simulink model "Motor_MapMdl_Ptbs_V1"  (R2018a)
settings: configuration reference "Config_Plant" (kept outside this file)
PreLoadFcn:
  | Motor_MapMdl_Ptbs_V1_BusInfo
model workspace (MAT data in the model file):
  mot.max_trq = 307
  mot.max_pwr = 124
  mot.spd = [0 500 1000 1500 2000 2500 3000 3500 3857.04487493 4000 4500 5000 5500 6000 6500 7000 7500 8000 8500 9000 9500 10000 10500 11000 11500 12000 12500]
  mot.trq = [307 307 307 307 307 307 307 307 307 296.028194151 263.136172579 236.822555321 215.29323211 197.352129434 182.171196401 169.158968086 157.881703547 148.014097075 139.307385483 131.568086289 124.643450169 118.41127766 112.772645391 107.646616055 102.9663284 98.676064717 94.7290221283]
  mot.trq_cp = [296.028194151 263.136172579 236.822555321 215.29323211 197.352129434 182.171196401 169.158968086 157.881703547 148.014097075 139.307385483 131.568086289 124.643450169 118.41127766 112.772645391 107.646616055 102.9663284 98.676064717 94.7290221283]
  mot.J = 0.02
  mot.damp = 0.0001
  mot.Tc = 0.0267
  mot.map.spdindex = [0 1000 2000 3000 3857 4000 5000 6000 7000 8000 9000 10000 11000 12000 12584]
  mot.map.trqindex = [10 25 50 75 100 125 150 175 200 225 250 275 300 307]
  mot.map.eff = [84  90  90  90  90  90  90  90  90  90  90  90  90  90  90; 84  90  93  95  95  95  96  95  95  95  95  93  93  93  93; 84  90  93  95  95  95  96  95  96  95  95  95  95  93  93; 84  90  93  95  95  95  96  96  96  95  95  95  95  93  93; 84  90  93  95  95  95  96  96  96  95  95  93  93  93  90; 84  88  90  93  93  95  95  96  95  95  95  93  93  93  90; 84  88  90  90  90  93  95  95  95  93  93  93  93  93  90; 84  88  90  90  90  90  93  93  93  93  93  93  93  93  90; 84  84  88  90  90  90  93  93  93  93  93  93  93  93  90; 84  84  88  90  90  90  90  93  93  93  93  93  93  93  90; 84  84  84  90  90  90  90  93  93  93  93  93  93  93  90; 84  84  84  88  90  90  90  93  93  93  93  93  93  93  90; 84  84  84  88  88  88  90  93  93  93  93  93  93  93  90; 84  84  84  88  88  88  90  93  93  93  93  93  93  93  90]
  mot.m = 30
  mot.Cp = 200
values from neighbouring files (symbols this model uses):
  mot = struct    [Motor_V1.m]
libraries: autolibmappedmotor x1
settings Model: Creator=IAEC Nishito  LastModifiedBy=E00026
settings ConfigSetRef: SourceLocation=Base Workspace

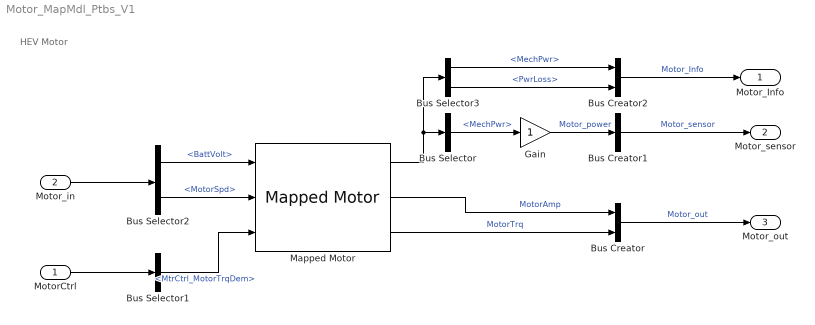
== system Motor_MapMdl_Ptbs_V1 ==
  note: HEV Motor
  MotorCtrl : Inport  OutDataTypeStr=Bus: MotorCtrl_Bus  SampleTime=0
      settings: AttributesFormatString=%<OutDataTypeStr>
  Motor_in : Inport  Port=2  OutDataTypeStr=Bus: Motor_in_Bus
      settings: AttributesFormatString=%<OutDataTypeStr>
  Bus Creator : BusCreator  Inputs=2  OutDataTypeStr=Bus: Motor_out_Bus
      settings: AttributesFormatString=%<OutDataTypeStr>
  Bus Creator1 : BusCreator  Inputs=1  OutDataTypeStr=Bus: Motor_sensor_Bus
      settings: AttributesFormatString=%<OutDataTypeStr>
  Bus Creator2 : BusCreator  Inputs=2  OutDataTypeStr=Bus: Motor_Info_out_Bus
      settings: AttributesFormatString=%<OutDataTypeStr>
  Bus Selector : BusSelector  OutputSignals=MechPwr
  Bus Selector1 : BusSelector  OutputSignals=MtrCtrl_MotorTrqDem
  Bus Selector2 : BusSelector  OutputSignals=BattVolt,MotorSpd
  Bus Selector3 : BusSelector  OutputSignals=MechPwr,PwrLoss
  Gain : Gain
  Mapped Motor : autolibmappedmotor/Mapped Motor  port_config=Speed  param_by=Maximum torque and power  w_t=[ 0 375 750 800 ]  T_t=[0.09 0.08 0.07 0]  torque_max=307  power_max=124e3  Tc=0.02  param_loss=Tabulated efficiency data  eff=100  w_eff=375  T_eff=0.08  Piron=0  Pbase=0  w_eff_bp=mot.map.spdindex.*pi/30  T_eff_bp=mot.map.trqindex  losses_table=[1 2;3 4]  efficiency_table=mot.map.eff'  J=5e-6  b=1e-5  omega_o=0  T_t_extended=[0 0.07 0.08 0.09 0.08 0.07 0]  w_t_extended=[-800 -750 -375 0 375 750 800]  KLossIron=0  KLossCopper=0  x_w_eff_vec=[-1317.7933984258 -1256.63706143592 -1151.91730631626 -1047.1975511966 -942.477796076938 -837.758040957278 -733.038285837618 -628.318530717959 -523.598775598299 -418.879020478639 -403.904095496528 -314.159265358979 -209.43951023932 -104.71975511966 0 104.71975511966 209.43951023932 314.159265358979 403.904095496528 418.879020478639 523.598775598299 628.318530717959 733.038285837618 837.758040957278 942.477796076938 1047.1975511966 1151.91730631626 1256.63706143592 1317.7933984258]  x_T_eff_vec=[-307 -300 -275 -250 -225 -200 -175 -150 -125 -100 -75 -50 -25 -10 10 25 50 75 100 125 150 175 200 225 250 275 300 307]  x_losses_mat=[44951.3970351912 43926.4466141933 40265.9093963439 36605.3721784944 32944.834960645 29284.2977427955 25623.7605249461 21963.2233070967 18302.6860892472 14642.1488713978 7439.15628143595 4959.4375209573 2479.71876047865 1464.21488713978 1317.7933984258 2306.13844724515 4612.27689449029 6918.41534173544 13177.933984258 16472.4174803225 19766.900976387 23061.3844724515 26355.867968516 29650.3514645805 32944.834960645 36239.3184567095 39533.801952774 40456.257331672;29037.7746776966 28375.675580811 26011.0359490768 23646.3963173425 21281.7566856083 18917.117053874 16552.4774221398 14187.8377904055 11823.1981586713 9458.558526937 7093.91889520275 4729.2792634685 2364.63963173425 1396.26340159546 1256.63706143592 2199.11485751285 4398.22971502571 6597.34457253856 8796.45943005141 10995.5742875643 13194.6891450771 15393.80400259 17592.9188601028 19792.0337176157 21991.1485751285 24190.2634326414 26389.3782901542 27005.1304502578;26617.9601212219 26011.0359490768 23843.449619987 21675.8632908973 19508.2769618076 17340.6906327178 15173.1043036281 13005.5179745384 10837.9316454486 8670.34531635892 4547.0419986168 3031.3613324112 2167.58632908973 1279.90811812918 1151.91730631626 2015.85528605345 2879.79326579064 4319.68989868596 8063.4211442138 10079.2764302672 12095.1317163207 14110.9870023741 16126.8422884276 18142.697574481 20158.5528605345 22174.4081465879 24190.2634326414 24754.7029127364;24198.1455647472 23646.3963173425 21675.8632908973 19705.3302644521 17734.7972380069 15764.2642115617 13793.7311851165 11823.1981586713 9852.66513222605 7882.13210578084 4133.67454419709 2755.78302946473 1970.53302644521 1163.55283466289 1047.1975511966 1832.59571459404 2617.99387799149 3926.99081698724 7330.38285837618 9162.97857297022 10995.5742875643 12828.1700021583 14660.7657167524 16493.3614313464 18325.9571459404 20158.5528605345 21991.1485751285 22504.2753752149;21778.3310082725 21281.7566856083 19508.2769618076 17734.7972380069 15961.3175142062 14187.8377904055 12414.3580666048 10640.8783428041 6200.51181629564 4960.40945303651 3720.30708977738 2480.20472651826 1240.10236325913 1047.1975511966 942.477796076938 1178.09724509617 2356.19449019234 3534.29173528851 4712.38898038468 5890.48622548085 9896.01685880784 11545.3530019425 13194.6891450771 14844.0252882118 16493.3614313464 18142.697574481 19792.0337176157 20253.8478376934;19358.5164517977 18917.117053874 17340.6906327178 15764.2642115617 14187.8377904055 12611.4113692493 11034.9849480932 9458.558526937 5511.56605892945 4409.25284714356 3306.93963535767 2204.62642357178 1102.31321178589 930.842267730309 837.758040957278 1047.1975511966 2094.39510239319 3141.59265358979 4188.79020478639 5235.98775598298 8796.45943005141 10262.5360017266 11728.6125734019 13194.6891450771 14660.7657167524 16126.8422884276 17592.9188601028 18003.4203001719;16938.701895323 16552.4774221398 15173.1043036281 13793.7311851165 12414.3580666048 11034.9849480932 9655.61182958152 5787.14436187593 4822.62030156327 3054.32619099008 2290.74464324256 1527.16309549504 964.524060312655 814.486984264021 733.038285837618 916.297857297022 1466.07657167524 2199.11485751286 2932.15314335048 4581.48928648511 5497.78714378213 8979.71900151082 10262.5360017266 11545.3530019425 12828.1700021583 14110.9870023741 15393.80400259 15752.9927626504;14518.8873388483 14187.8377904055 13005.5179745384 11823.1981586713 10640.8783428041 9458.558526937 8276.23871106988 4960.40945303651 3272.49234748937 2617.9938779915 1963.49540849362 1653.46981767884 826.734908839418 698.131700797732 628.318530717959 785.398163397447 1570.79632679489 1884.95559215388 2513.27412287184 3141.5926535898 4712.38898038468 7696.90200129499 8796.45943005141 9896.01685880784 10995.5742875643 12095.1317163207 13194.6891450771 13502.5652251289;17860.5360120753 17453.2925199433 15998.8514766147 14544.4104332861 13089.9693899575 7882.13210578084 6896.86559255823 4133.67454419709 3444.72878683091 2181.66156499292 1636.24617374469 1090.83078249646 545.415391248229 ...(+9284 chars)]  aMode=aMode
      settings: SourceProductName=Powertrain Blockset  SourceProductBaseCode=PW
  Motor_Info : Outport  OutDataTypeStr=Bus: Motor_Info_out_Bus
      settings: AttributesFormatString=%<OutDataTypeStr>
  Motor_sensor : Outport  Port=2  OutDataTypeStr=Bus: Motor_sensor_Bus
      settings: AttributesFormatString=%<OutDataTypeStr>
  Motor_out : Outport  Port=3  OutDataTypeStr=Bus: Motor_out_Bus
      settings: AttributesFormatString=%<OutDataTypeStr>
  wires:
  Mapped Motor/2 -> Bus Creator/1  "MotorAmp"
  Mapped Motor/1 -> Bus Selector3/1, Bus Selector/1
  Mapped Motor/3 -> Bus Creator/2  "MotorTrq"
  Bus Creator1/1 -> Motor_sensor/1  "Motor_sensor"
  Bus Selector/1 -> Gain/1  "<MechPwr>"
  Gain/1 -> Bus Creator1/1  "Motor_power"
  Bus Selector1/1 -> Mapped Motor/3  "<MtrCtrl_MotorTrqDem>"
  Bus Creator/1 -> Motor_out/1  "Motor_out"
  Bus Selector2/1 -> Mapped Motor/1  "<BattVolt>"
  Bus Selector2/2 -> Mapped Motor/2  "<MotorSpd>"
  Motor_in/1 -> Bus Selector2/1
  MotorCtrl/1 -> Bus Selector1/1
  Bus Selector3/1 -> Bus Creator2/1  "<MechPwr>"
  Bus Selector3/2 -> Bus Creator2/2  "<PwrLoss>"
  Bus Creator2/1 -> Motor_Info/1  "Motor_Info"
